simulink model "problem1"  (R2024b)
settings: Solver=VariableStepAuto  StartTime=0.0  StopTime=100  RelTol=1e-3
model workspace (MAT data in the model file):
  a_m = 0.7408
  b_m = 0.2592
settings Model: Creator=djd14  LastModifiedBy=djd14

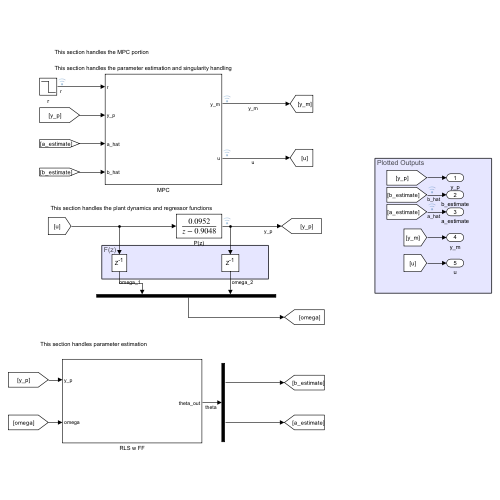
[thumbnail: Simulink's stored preview of the top-level diagram]
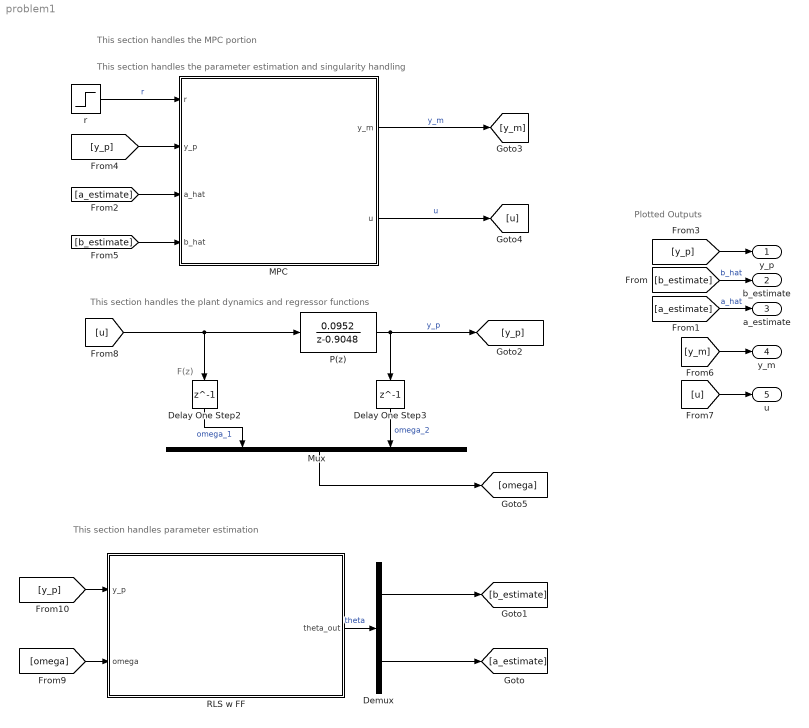
== system problem1 ==
  note: This section handles parameter estimation
  note: This section handles the parameter estimation and singularity handling
  note: This section handles the plant dynamics and regressor functions
  note: This section handles the MPC portion
  note: Plotted Outputs
  note: F(z)
  Delay One Step2 : Delay  DelayLength=1
  Delay One Step3 : Delay  DelayLength=1
  Demux : Demux  Outputs=2
  MPC : Subsystem
  Mux : Mux  Inputs=2
  P(z) : DiscreteTransferFcn  Numerator=[0.0952]  Denominator=[1 -0.9048]
  RLS w FF : Subsystem
  r : Step  Time=50  Before=1  After=-1  SampleTime=0
  y_p : Outport  SampleTime=1
  b_estimate : Outport  Port=2
  a_estimate : Outport  Port=3
  y_m : Outport  Port=4
  u : Outport  Port=5
  wires:
  Delay One Step3/1 -> Mux/2  "omega_2"
  Delay One Step2/1 -> Mux/1  "omega_1"
  RLS w FF/1(theta_out) -> Demux/1  "theta"
  Mux/1 -> [omega]
  P(z)/1 -> [y_p], Delay One Step3/1  "y_p"
  Demux/2 -> [a_estimate]
  [b_estimate] -> b_estimate/1  "b_hat"
  [a_estimate] -> a_estimate/1  "a_hat"
  r/1 -> MPC/1(r)  "r"
  [y_p] -> y_p/1
  [b_estimate] -> MPC/4(b_hat)
  [a_estimate] -> MPC/3(a_hat)
  [y_p] -> MPC/2(y_p)
  MPC/1(y_m) -> [y_m]  "y_m"
  MPC/2(u) -> [u]  "u"
  [y_m] -> y_m/1
  [u] -> u/1
  [u] -> P(z)/1, Delay One Step2/1
  [omega] -> RLS w FF/2(omega)
  [y_p] -> RLS w FF/1(y_p)
  Demux/1 -> [b_estimate]

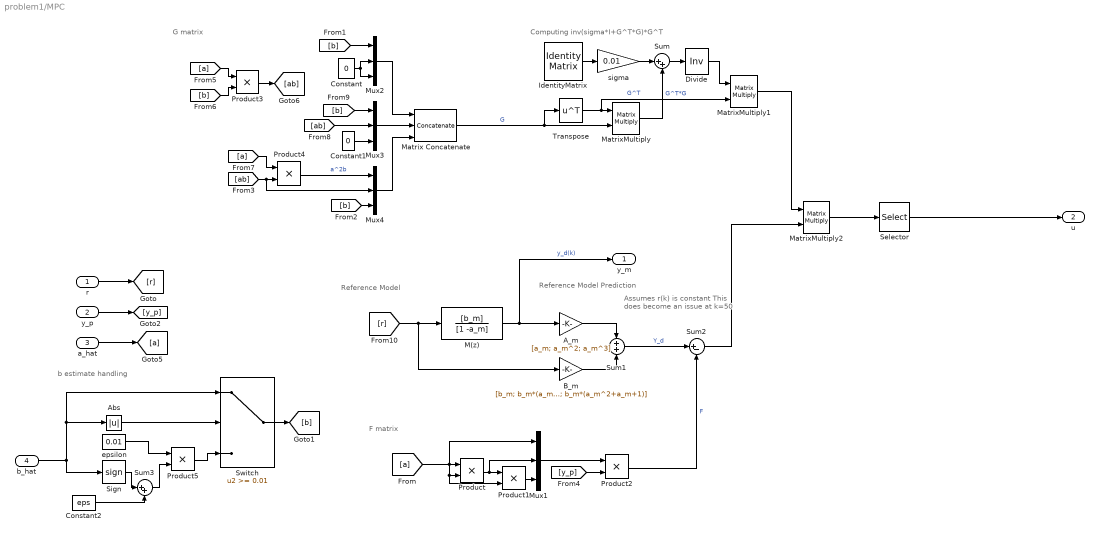
== system problem1/MPC ==
  note: Assumes r(k) is constant
      | This does become an issue at k=50
  note: Reference Model Prediction
  note: Reference Model
  note: Computing inv(sigma*I+G^T*G)*G^T
  note: G matrix
  note: F matrix
  note: b estimate handling
  r : Inport
  y_p : Inport  Port=2
  a_hat : Inport  Port=3
  b_hat : Inport  Port=4
  A_m : Gain  Gain=[a_m; a_m^2; a_m^3]
  Abs : Abs  SaturateOnIntegerOverflow=off
  B_m : Gain  Gain=[b_m; b_m*(a_m+1); b_m*(a_m^2+a_m+1)]
  Constant : Constant  Value=0
  Constant1 : Constant  Value=0
  Constant2 : Constant  Value=eps
  Divide : Product  Inputs=/  Multiplication=Matrix(*)
  IdentityMatrix : IdentityMatrix  OutputDimensions=3
  M(z) : DiscreteTransferFcn  Numerator=[b_m]  Denominator=[1 -a_m]
  Matrix Concatenate : Concatenate  NumInputs=3  Mode=Multidimensional array  ConcatenateDimension=2
  MatrixMultiply : Product  Multiplication=Matrix(*)
  MatrixMultiply1 : Product  Multiplication=Matrix(*)
  MatrixMultiply2 : Product  Multiplication=Matrix(*)
  Mux{1..4} (4 alike) : Mux  Inputs=3
  Product{,1..5} (6 alike) : Product
  Selector : Selector  InputPortWidth=3  IndexOptions=Index vector (dialog)  Indices=[1]  OutputSizes=1
  Sign : Signum  ZeroCross=off
  Sum : Sum  Inputs=|++
  Sum1 : Sum  Inputs=+|+
  Sum2 : Sum  Inputs=|+-
  Sum3 : Sum  Inputs=|++
  Switch : Switch  Threshold=0.01  SaturateOnIntegerOverflow=off  InputSameDT=off
  Transpose : Math  Operator=transpose
  epsilon : Constant  Value=0.01
  sigma : Gain  Gain=0.01
  y_m : Outport
  u : Outport  Port=2
  wires:
  [a] -> Mux1/1, Product1/2, Product/2, Product/1
  [y_p] -> Product2/2
  Mux2/1 -> Matrix Concatenate/1
  Product1/1 -> Mux1/3
  [a] -> Product3/1
  Constant1/1 -> Mux3/3
  Product/1 -> Mux1/2, Product1/1
  Mux1/1 -> Product2/1
  Constant/1 -> Mux2/2, Mux2/3
  Matrix Concatenate/1 -> MatrixMultiply/2, Transpose/1  "G"
  Product2/1 -> Sum2/2  "F"
  Mux3/1 -> Matrix Concatenate/2
  Mux4/1 -> Matrix Concatenate/3
  [b] -> Mux2/1
  [b] -> Mux3/1
  [b] -> Mux4/3
  [b] -> Product3/2
  Product3/1 -> [ab]
  [ab] -> Product4/2, Mux4/2
  [a] -> Product4/1
  Product4/1 -> Mux4/1  "a^2b"
  [ab] -> Mux3/2
  IdentityMatrix/1 -> sigma/1
  sigma/1 -> Sum/1
  Transpose/1 -> MatrixMultiply1/2, MatrixMultiply/1  "G^T"
  Sum/1 -> Divide/1
  MatrixMultiply/1 -> Sum/2  "G^T*G"
  [r] -> B_m/1, M(z)/1
  M(z)/1 -> A_m/1, y_m/1  "y_d(k)"
  r/1 -> [r]
  a_hat/1 -> [a]
  y_p/1 -> [y_p]
  Sum1/1 -> Sum2/1  "Y_d"
  MatrixMultiply2/1 -> Selector/1
  MatrixMultiply1/1 -> MatrixMultiply2/1
  Sum2/1 -> MatrixMultiply2/2
  Divide/1 -> MatrixMultiply1/1
  Selector/1 -> u/1
  Switch/1 -> [b]
  Sign/1 -> Sum3/1
  epsilon/1 -> Product5/1
  Abs/1 -> Switch/2
  b_hat/1 -> Sign/1, Switch/1, Abs/1
  Product5/1 -> Switch/3
  Sum3/1 -> Product5/2
  Constant2/1 -> Sum3/2
  B_m/1 -> Sum1/2
  A_m/1 -> Sum1/1

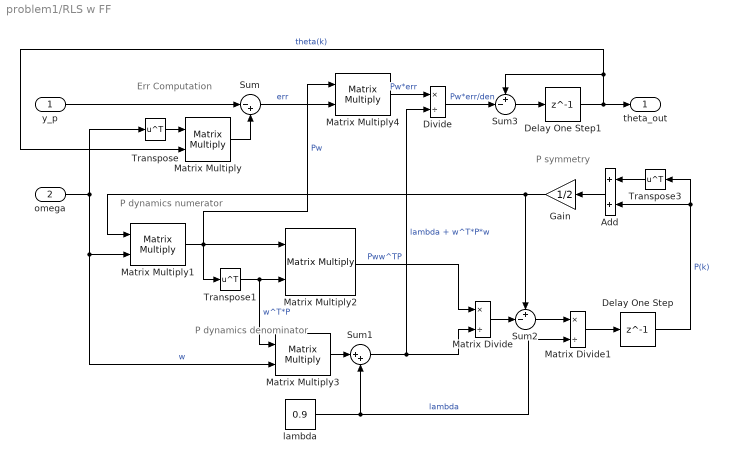
== system problem1/RLS w FF ==
  note: P symmetry
  note: P dynamics denominator
  note: P dynamics numerator
  note: Err Computation
  y_p : Inport
  omega : Inport  Port=2
  Add : Sum
  Delay One Step : Delay  DelayLength=1  InitialCondition=100*eye(2)
  Delay One Step1 : Delay  DelayLength=1  InitialCondition=[0 0]
  Divide : Product  Inputs=*/
  Gain : Gain  Gain=1/2
  Matrix Divide : Product  Inputs=*/
  Matrix Divide1 : Product  Inputs=*/
  Matrix Multiply{,1..4} (5 alike) : Product  Multiplication=Matrix(*)
  Sum : Sum  Inputs=|-+
  Sum1 : Sum  Inputs=|++
  Sum2 : Sum  Inputs=+-|
  Sum3 : Sum  Inputs=+-|
  Transpose : Math  Operator=transpose
  Transpose1 : Math  Operator=transpose
  Transpose3 : Math  Operator=transpose
  lambda : Constant  Value=0.9
  theta_out : Outport
  wires:
  omega/1 -> Transpose/1, Matrix Multiply3/2, Matrix Multiply1/2  "w"
  Transpose/1 -> Matrix Multiply/1
  y_p/1 -> Sum/1
  Matrix Multiply/1 -> Sum/2
  Sum/1 -> Matrix Multiply4/2  "err"
  Matrix Multiply1/1 -> Matrix Multiply4/1, Matrix Multiply2/1, Transpose1/1  "Pw"
  Delay One Step/1 -> Transpose3/1, Add/2  "P(k)"
  Matrix Multiply2/1 -> Matrix Divide/1  "Pww^TP"
  Transpose1/1 -> Matrix Multiply3/1, Matrix Multiply2/2  "w^T*P"
  Matrix Multiply3/1 -> Sum1/1
  Sum1/1 -> Divide/2, Matrix Divide/2  "lambda + w^T*P*w"
  Matrix Divide/1 -> Sum2/2
  Sum2/1 -> Matrix Divide1/1
  Matrix Divide1/1 -> Delay One Step/1
  Transpose3/1 -> Add/1
  Add/1 -> Gain/1
  Gain/1 -> Matrix Multiply1/1, Sum2/1
  lambda/1 -> Matrix Divide1/2, Sum1/2  "lambda"
  Sum3/1 -> Delay One Step1/1
  Delay One Step1/1 -> theta_out/1, Matrix Multiply/2, Sum3/1  "theta(k)"
  Matrix Multiply4/1 -> Divide/1  "Pw*err"
  Divide/1 -> Sum3/2  "Pw*err/den"
